simulink model "HelloWorldFig"  (Simulink 7.1)
settings: Solver=ode45  StartTime=0.0  StopTime=10.0  RelTol=1e-3
undefined symbols (not defined in the file): uk, xk
libraries: MPCMdlLib x9
settings Model: Creator=serg  LastModifiedBy=serg

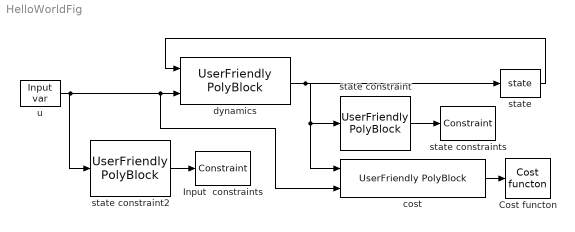
== system HelloWorldFig ==
  Cost functon : MPCMdlLib/Cost functon  Tag=OptCost
  Input  constraints : MPCMdlLib/Constraint  Tag=InequalBlock  CompareSign=< 0
  "cost " : MPCMdlLib/UserFriendly PolyBlock  Tag=PolyBlock  A=[2 0; 0 2]  C=[0.5 2]  gA=[0 0 ]  gC=1  input_type=Scalar  output_type=Scalar  port_names=xk,uk
  dynamics : MPCMdlLib/UserFriendly PolyBlock  Tag=PolyBlock  A=[1 0; 0 1]  C=[0.9 1]  gA=[0 0 ]  gC=1  input_type=Scalar  output_type=Scalar  port_names=xk,uk
  state : MPCMdlLib/state  Tag=OptState  SystemSampleTime=-1  init_val=1  save_name=BL_System_state
  state constraint : MPCMdlLib/UserFriendly PolyBlock  Tag=PolyBlock  A="[1  ;  0 ]"  C=[1 -1 ; -1 0.5 ]  gA="[0  ]"  gC=1  input_type=Scalar  output_type=Vector  port_names=x
  state constraint2 : MPCMdlLib/UserFriendly PolyBlock  Tag=PolyBlock  A="[1  ;  0 ]"  C=[1 -2 ; -1 -2 ]  gA="[0  ]"  gC=1  input_type=Scalar  output_type=Vector  port_names=u
  state constraints : MPCMdlLib/Constraint  Tag=InequalBlock  CompareSign=< 0
  u : MPCMdlLib/Input var  Tag=OptInput  SystemSampleTime=-1  step_ratio=1  save_name=BL_System_u
  wires:
  dynamics/1 -> state/1, "cost "/1, state constraint/1
  state/1 -> dynamics/1
  u/1 -> dynamics/2, "cost "/2, state constraint2/1
  "cost "/1 -> Cost functon/1
  state constraint/1 -> state constraints/1
  state constraint2/1 -> Input  constraints/1
